simulink model "LVLH_Attitude_for_EquatorialOrbit"  (R2018b)
settings: Solver=VariableStepAuto  StartTime=0.0  StopTime=43200  RelTol=1e-3
libraries: simulink x2, shared6dof x1, vrlib x1
settings Model: Creator=Victor  LastModifiedBy=Victor

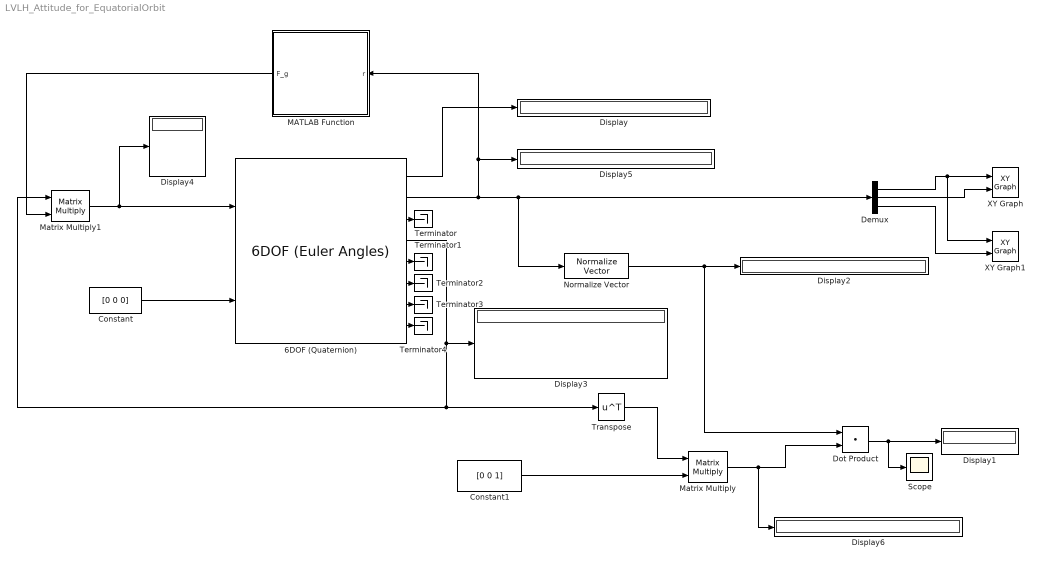
== system LVLH_Attitude_for_EquatorialOrbit ==
  6DOF (Quaternion) : shared6dof/6DOF (Euler Angles)  units=Metric (MKS)  mtype=Fixed  rep=Quaternion  xme_0=r_ECI  Vm_0=v_B  eul_0=Eu  pm_0=w  mass_0=1.0  mass_e=0.5  mass_f=2.0  inertia=eye(3)  inertia_e=eye(3)  inertia_f=2*eye(3)  k_quat=1.0  vre_flag=on  abi_flag=off  aMode=0  xme_statename=''  Vm_statename=''  eul_statename=''  quat_statename=''  pm_statename=''  mass_statename=''
      settings: SourceProductBaseCode=AE
  Constant : Constant  Value=[0 0 0]
  Constant1 : Constant  Value=[0 0 1]
  Demux : Demux  Outputs=3
  Display{,1..6} (7 alike) : Display
  Dot Product : DotProduct  InputSameDT=on  OutDataTypeStr=Inherit: Inherit via internal rule
  MATLAB Function : MATLAB Function  TreatAsAtomicUnit=on
  Matrix Multiply : Product  Multiplication=Matrix(*)
  Matrix Multiply1 : Product  Multiplication=Matrix(*)
  Normalize Vector : vrlib/Utilities/Normalize Vector  maxzero=0
      settings: SourceProductName=Simulink 3D Animation  SourceProductBaseCode=VR
  Scope : Scope
  Terminator{,1..4} (5 alike) : Terminator
  Transpose : Math  Operator=transpose  SaturateOnIntegerOverflow=on
  XY Graph : simulink/Sinks/XY Graph  xmin=-1  xmax=1  ymin=-1  ymax=1  st=-1
  XY Graph1 : simulink/Sinks/XY Graph  xmin=-15000  xmax=15000  ymin=-15000  ymax=15000  st=0
  wires:
  6DOF (Quaternion)/2 -> Display5/1, MATLAB Function/1(r), Normalize Vector/1, Demux/1
  Constant/1 -> 6DOF (Quaternion)/2
  6DOF (Quaternion)/1 -> Display/1
  6DOF (Quaternion)/4 -> Display3/1, Transpose/1, Matrix Multiply1/1
  Constant1/1 -> Matrix Multiply/2
  Normalize Vector/1 -> Dot Product/1, Display2/1
  Dot Product/1 -> Display1/1, Scope/1
  Demux/1 -> XY Graph/1, XY Graph1/1
  Demux/2 -> XY Graph/2
  Demux/3 -> XY Graph1/2
  Transpose/1 -> Matrix Multiply/1
  Matrix Multiply/1 -> Display6/1, Dot Product/2
  Matrix Multiply1/1 -> Display4/1, 6DOF (Quaternion)/1
  MATLAB Function/1(F_g) -> Matrix Multiply1/2
  6DOF (Quaternion)/3 -> Terminator/1
  6DOF (Quaternion)/5 -> Terminator1/1
  6DOF (Quaternion)/6 -> Terminator2/1
  6DOF (Quaternion)/7 -> Terminator3/1
  6DOF (Quaternion)/8 -> Terminator4/1

== matlab function LVLH_Attitude_for_EquatorialOrbit/MATLAB Function ==
  data: r input; F_g output
function F_g = OrbitDynamics(r)

mu = 3.986*10^5;%km^3/sec^2
F_g = -mu/norm(r)^3*r;
